simulink model "TR_Plausability"  (R2024b)
settings: Solver=VariableStepAuto  StartTime=0.0  StopTime=25  RelTol=1e-3
libraries: simulink x2
settings Model: Creator=feder  LastModifiedBy=Michele
settings ConfigComp: CovMetricSettings=dcmwe

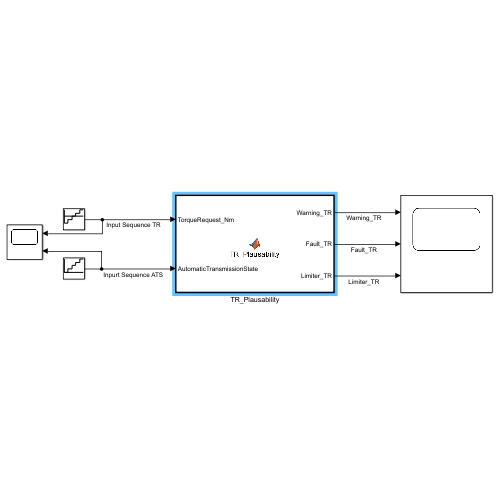
[thumbnail: Simulink's stored preview of the top-level diagram]
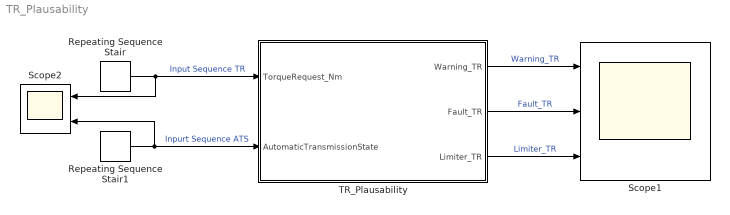
== system TR_Plausability ==
  Repeating Sequence Stair : simulink/Sources/Repeating Sequence Stair  OutValues=[-90 -45 0 45 90].'  tsamp=1  OutMin=[]  OutMax=[]  OutDataTypeStr=single  OutputDataTypeScalingMode=single  OutDataType=Enum: TransmissionState  ConRadixGroup=Best Precision: Vector-wise  OutScaling=[]
  Repeating Sequence Stair1 : simulink/Sources/Repeating Sequence Stair  OutValues=[0 1 2 3 4].'  tsamp=5  OutMin=[]  OutMax=[]  OutDataTypeStr=single  OutputDataTypeScalingMode=single  OutDataType=Enum: TransmissionState  ConRadixGroup=Best Precision: Vector-wise  OutScaling=[]
  Scope1 : Scope  NumInputPorts=3
  Scope2 : Scope  NumInputPorts=2
  TR_Plausability : MATLAB Function  TreatAsAtomicUnit=on
  wires:
  Repeating Sequence Stair/1 -> Scope2/1, TR_Plausability/1(TorqueRequest_Nm)  "Input Sequence TR"
  TR_Plausability/3(Limiter_TR) -> Scope1/3  "Limiter_TR"
  TR_Plausability/1(Warning_TR) -> Scope1/1  "Warning_TR"
  Repeating Sequence Stair1/1 -> Scope2/2, TR_Plausability/2(AutomaticTransmissionState)  "Inpurt Sequence ATS"
  TR_Plausability/2(Fault_TR) -> Scope1/2  "Fault_TR"

== matlab function TR_Plausability/TR_Plausability ==
  data: Warning_TR output Enum: WarningType; TorqueRequest_Nm input single; Fault_TR output boolean; AutomaticTransmissionState input; Limiter_TR output boolean
function [Warning_TR,Fault_TR,Limiter_TR] = TR_Plausability(TorqueRequest_Nm,AutomaticTransmissionState)

Warning_TR = WarningType(0);
Fault_TR = boolean(0);
Limiter_TR = boolean(0);

PositiveMode = [TransmissionState.Drive, TransmissionState.Brake];
NegativeMode = [TransmissionState.Reverse, TransmissionState.Brake];

if ((TorqueRequest_Nm == 0 ) ...
        || (TorqueRequest_Nm > 0 && any(AutomaticTransmissionState == PositiveMode)) ...
        || (TorqueRequest_Nm < 0  && any(AutomaticTransmissionState == NegativeMode)))
    
    if (TorqueRequest_Nm > 80 || TorqueRequest_Nm < -80 )
        
        Warning_TR =  WarningType(1);
        Limiter_TR = boolean(1);
        
    end

else

    Warning_TR =  WarningType(2);
    Fault_TR = boolean(1); 

end
